simulink model "VCU_CS75_12_16_Test"  (R2014a)
settings: Solver=FixedStepDiscrete  StartTime=0.0  StopTime=25  FixedStep=0.0005  RelTol=1e-3
undefined symbols (not defined in the file): ecucoder_acal, I_SW01_L, LaterlAngleCommand, LDW, RemoteAcclPosition
libraries: simulink x913, ec5744lib x39
(part 30 of 30)

== system VCU_CS75_12_16_Test/长安CS75底盘程序，20ms一次/Input/CAN1_Rx/ESP_277/ReceiveMessages/Subsystem/ESP_1/ESP_AWBavailable_Sub ==
  In1 : Inport
  Out1 : Outport
  wires:
  In1/1 -> Out1/1

== system VCU_CS75_12_16_Test/长安CS75底盘程序，20ms一次/Input/CAN1_Rx/ESP_277/ReceiveMessages/Subsystem/ESP_1/ESP_BrakeForce_Sub ==
  In1 : Inport
  Out1 : Outport
  wires:
  In1/1 -> Out1/1

== system VCU_CS75_12_16_Test/长安CS75底盘程序，20ms一次/Input/CAN1_Rx/ESP_277/ReceiveMessages/Subsystem/ESP_1/ESP_BrakeOverHeat_Sub ==
  In1 : Inport
  Out1 : Outport
  wires:
  In1/1 -> Out1/1

== system VCU_CS75_12_16_Test/长安CS75底盘程序，20ms一次/Input/CAN1_Rx/ESP_277/ReceiveMessages/Subsystem/ESP_1/ESP_CDD_Active_APA_Sub ==
  In1 : Inport
  Out1 : Outport
  wires:
  In1/1 -> Out1/1

== system VCU_CS75_12_16_Test/长安CS75底盘程序，20ms一次/Input/CAN1_Rx/ESP_277/ReceiveMessages/Subsystem/ESP_1/ESP_CDD_Active_Sub ==
  In1 : Inport
  Out1 : Outport
  wires:
  In1/1 -> Out1/1

== system VCU_CS75_12_16_Test/长安CS75底盘程序，20ms一次/Input/CAN1_Rx/ESP_277/ReceiveMessages/Subsystem/ESP_1/ESP_CDD_Available_APA_Sub ==
  In1 : Inport
  Out1 : Outport
  wires:
  In1/1 -> Out1/1

== system VCU_CS75_12_16_Test/长安CS75底盘程序，20ms一次/Input/CAN1_Rx/ESP_277/ReceiveMessages/Subsystem/ESP_1/ESP_CDD_Available_Sub ==
  In1 : Inport
  Out1 : Outport
  wires:
  In1/1 -> Out1/1

== system VCU_CS75_12_16_Test/长安CS75底盘程序，20ms一次/Input/CAN1_Rx/ESP_277/ReceiveMessages/Subsystem/ESP_1/ESP_CheckSum_277_Sub ==
  In1 : Inport
  Out1 : Outport
  wires:
  In1/1 -> Out1/1

== system VCU_CS75_12_16_Test/长安CS75底盘程序，20ms一次/Input/CAN1_Rx/ESP_277/ReceiveMessages/Subsystem/ESP_1/ESP_PrefillActive_Sub ==
  In1 : Inport
  Out1 : Outport
  wires:
  In1/1 -> Out1/1

== system VCU_CS75_12_16_Test/长安CS75底盘程序，20ms一次/Input/CAN1_Rx/ESP_277/ReceiveMessages/Subsystem/ESP_1/ESP_PrefillAvailable_Sub ==
  In1 : Inport
  Out1 : Outport
  wires:
  In1/1 -> Out1/1

== system VCU_CS75_12_16_Test/长安CS75底盘程序，20ms一次/Input/CAN1_Rx/ESP_277/ReceiveMessages/Subsystem/ESP_1/ESP_RollingCounter_277_Sub ==
  In1 : Inport
  Out1 : Outport
  wires:
  In1/1 -> Out1/1

== system VCU_CS75_12_16_Test/长安CS75底盘程序，20ms一次/Input/CAN1_Rx/ESP_277/ReceiveMessages/Subsystem/ESP_1/ESP_TCSActive_Sub ==
  In1 : Inport
  Out1 : Outport
  wires:
  In1/1 -> Out1/1

== system VCU_CS75_12_16_Test/长安CS75底盘程序，20ms一次/Input/CAN1_Rx/ESP_277/ReceiveMessages/Subsystem/ESP_1/ESP_VDCActive_Sub ==
  In1 : Inport
  Out1 : Outport
  wires:
  In1/1 -> Out1/1

== system VCU_CS75_12_16_Test/长安CS75底盘程序，20ms一次/Input/CAN1_Rx/ESP_277/ReceiveMessages/Subsystem/ESP_1/ESP_VehicleStandstill_Sub ==
  In1 : Inport
  Out1 : Outport
  wires:
  In1/1 -> Out1/1

== system VCU_CS75_12_16_Test/长安CS75底盘程序，20ms一次/Input/CAN1_Rx/ESP_280/ReceiveMessages/Subsystem/ESP_1/Wheel_Speed_FL_Data_Sub ==
  In1 : Inport
  Out1 : Outport
  wires:
  In1/1 -> Out1/1

== system VCU_CS75_12_16_Test/长安CS75底盘程序，20ms一次/Input/CAN1_Rx/ESP_280/ReceiveMessages/Subsystem/ESP_1/Wheel_Speed_FL_Direction_Sub ==
  In1 : Inport
  Out1 : Outport
  wires:
  In1/1 -> Out1/1

== system VCU_CS75_12_16_Test/长安CS75底盘程序，20ms一次/Input/CAN1_Rx/ESP_280/ReceiveMessages/Subsystem/ESP_1/Wheel_Speed_FL_Valid_Data_Sub ==
  In1 : Inport
  Out1 : Outport
  wires:
  In1/1 -> Out1/1

== system VCU_CS75_12_16_Test/长安CS75底盘程序，20ms一次/Input/CAN1_Rx/ESP_280/ReceiveMessages/Subsystem/ESP_1/Wheel_Speed_FR_Data_Sub ==
  In1 : Inport
  Out1 : Outport
  wires:
  In1/1 -> Out1/1

== system VCU_CS75_12_16_Test/长安CS75底盘程序，20ms一次/Input/CAN1_Rx/ESP_280/ReceiveMessages/Subsystem/ESP_1/Wheel_Speed_FR_Direction_Sub ==
  In1 : Inport
  Out1 : Outport
  wires:
  In1/1 -> Out1/1

== system VCU_CS75_12_16_Test/长安CS75底盘程序，20ms一次/Input/CAN1_Rx/ESP_280/ReceiveMessages/Subsystem/ESP_1/Wheel_Speed_FR_Valid_Data_Sub ==
  In1 : Inport
  Out1 : Outport
  wires:
  In1/1 -> Out1/1

== system VCU_CS75_12_16_Test/长安CS75底盘程序，20ms一次/Input/CAN1_Rx/ESP_280/ReceiveMessages/Subsystem/ESP_1/Wheel_Speed_RL_Data_Sub ==
  In1 : Inport
  Out1 : Outport
  wires:
  In1/1 -> Out1/1

== system VCU_CS75_12_16_Test/长安CS75底盘程序，20ms一次/Input/CAN1_Rx/ESP_280/ReceiveMessages/Subsystem/ESP_1/Wheel_Speed_RL_Direction_Sub ==
  In1 : Inport
  Out1 : Outport
  wires:
  In1/1 -> Out1/1

== system VCU_CS75_12_16_Test/长安CS75底盘程序，20ms一次/Input/CAN1_Rx/ESP_280/ReceiveMessages/Subsystem/ESP_1/Wheel_Speed_RL_Valid_Data_Sub ==
  In1 : Inport
  Out1 : Outport
  wires:
  In1/1 -> Out1/1

== system VCU_CS75_12_16_Test/长安CS75底盘程序，20ms一次/Input/CAN1_Rx/ESP_280/ReceiveMessages/Subsystem/ESP_1/Wheel_Speed_RR_Data_Sub ==
  In1 : Inport
  Out1 : Outport
  wires:
  In1/1 -> Out1/1

== system VCU_CS75_12_16_Test/长安CS75底盘程序，20ms一次/Input/CAN1_Rx/ESP_280/ReceiveMessages/Subsystem/ESP_1/Wheel_Speed_RR_Direction_Sub ==
  In1 : Inport
  Out1 : Outport
  wires:
  In1/1 -> Out1/1

== system VCU_CS75_12_16_Test/长安CS75底盘程序，20ms一次/Input/CAN1_Rx/ESP_280/ReceiveMessages/Subsystem/ESP_1/Wheel_Speed_RR_Valid_Data_Sub ==
  In1 : Inport
  Out1 : Outport
  wires:
  In1/1 -> Out1/1

== system VCU_CS75_12_16_Test/长安CS75底盘程序，20ms一次/Input/CAN1_Rx/ESP_281/ReceiveMessages/Subsystem/ESP_2/ESP_ABSActiveStatus_Sub ==
  In1 : Inport
  Out1 : Outport
  wires:
  In1/1 -> Out1/1

== system VCU_CS75_12_16_Test/长安CS75底盘程序，20ms一次/Input/CAN1_Rx/ESP_281/ReceiveMessages/Subsystem/ESP_2/ESP_ABSFailStatus_Sub ==
  In1 : Inport
  Out1 : Outport
  wires:
  In1/1 -> Out1/1

== system VCU_CS75_12_16_Test/长安CS75底盘程序，20ms一次/Input/CAN1_Rx/ESP_281/ReceiveMessages/Subsystem/ESP_2/ESP_BrakePedalStatus_Sub ==
  In1 : Inport
  Out1 : Outport
  wires:
  In1/1 -> Out1/1

== system VCU_CS75_12_16_Test/长安CS75底盘程序，20ms一次/Input/CAN1_Rx/ESP_281/ReceiveMessages/Subsystem/ESP_2/ESP_Checksum_Sub ==
  In1 : Inport
  Out1 : Outport
  wires:
  In1/1 -> Out1/1

== system VCU_CS75_12_16_Test/长安CS75底盘程序，20ms一次/Input/CAN1_Rx/ESP_281/ReceiveMessages/Subsystem/ESP_2/ESP_EBDFailStatus_Sub ==
  In1 : Inport
  Out1 : Outport
  wires:
  In1/1 -> Out1/1

== system VCU_CS75_12_16_Test/长安CS75底盘程序，20ms一次/Input/CAN1_Rx/ESP_281/ReceiveMessages/Subsystem/ESP_2/ESP_ESPActiveStatus_Sub ==
  In1 : Inport
  Out1 : Outport
  wires:
  In1/1 -> Out1/1

== system VCU_CS75_12_16_Test/长安CS75底盘程序，20ms一次/Input/CAN1_Rx/ESP_281/ReceiveMessages/Subsystem/ESP_2/ESP_ESPFailStatus_Sub ==
  In1 : Inport
  Out1 : Outport
  wires:
  In1/1 -> Out1/1

== system VCU_CS75_12_16_Test/长安CS75底盘程序，20ms一次/Input/CAN1_Rx/ESP_281/ReceiveMessages/Subsystem/ESP_2/ESP_ESPSwitchStatus_Sub ==
  In1 : Inport
  Out1 : Outport
  wires:
  In1/1 -> Out1/1

== system VCU_CS75_12_16_Test/长安CS75底盘程序，20ms一次/Input/CAN1_Rx/ESP_281/ReceiveMessages/Subsystem/ESP_2/ESP_RollingCounter_Sub ==
  In1 : Inport
  Out1 : Outport
  wires:
  In1/1 -> Out1/1

== system VCU_CS75_12_16_Test/长安CS75底盘程序，20ms一次/Input/CAN1_Rx/ESP_281/ReceiveMessages/Subsystem/ESP_2/ESP_VehicleSpeed_Status_Sub ==
  In1 : Inport
  Out1 : Outport
  wires:
  In1/1 -> Out1/1

== system VCU_CS75_12_16_Test/长安CS75底盘程序，20ms一次/Input/CAN1_Rx/ESP_281/ReceiveMessages/Subsystem/ESP_2/ESP_VehicleSpeed_Sub ==
  In1 : Inport
  Out1 : Outport
  wires:
  In1/1 -> Out1/1

== system VCU_CS75_12_16_Test/长安CS75底盘程序，20ms一次/Input/CAN1_Rx/ESP_287/ReceiveMessages/Subsystem/ESP_2/ESP_CheckSum_Sub ==
  In1 : Inport
  Out1 : Outport
  wires:
  In1/1 -> Out1/1

== system VCU_CS75_12_16_Test/长安CS75底盘程序，20ms一次/Input/CAN1_Rx/ESP_287/ReceiveMessages/Subsystem/ESP_2/ESP_HBBActiveStatus_Sub ==
  In1 : Inport
  Out1 : Outport
  wires:
  In1/1 -> Out1/1

== system VCU_CS75_12_16_Test/长安CS75底盘程序，20ms一次/Input/CAN1_Rx/ESP_287/ReceiveMessages/Subsystem/ESP_2/ESP_HBB_Status_Sub ==
  In1 : Inport
  Out1 : Outport
  wires:
  In1/1 -> Out1/1

== system VCU_CS75_12_16_Test/长安CS75底盘程序，20ms一次/Input/CAN1_Rx/ESP_287/ReceiveMessages/Subsystem/ESP_2/ESP_HDC_Status_Sub ==
  In1 : Inport
  Out1 : Outport
  wires:
  In1/1 -> Out1/1

== system VCU_CS75_12_16_Test/长安CS75底盘程序，20ms一次/Input/CAN1_Rx/ESP_287/ReceiveMessages/Subsystem/ESP_2/ESP_HHC_Available_Sub ==
  In1 : Inport
  Out1 : Outport
  wires:
  In1/1 -> Out1/1

== system VCU_CS75_12_16_Test/长安CS75底盘程序，20ms一次/Input/CAN1_Rx/ESP_287/ReceiveMessages/Subsystem/ESP_2/ESP_LatAcceleration_Sub ==
  In1 : Inport
  Out1 : Outport
  wires:
  In1/1 -> Out1/1

== system VCU_CS75_12_16_Test/长安CS75底盘程序，20ms一次/Input/CAN1_Rx/ESP_287/ReceiveMessages/Subsystem/ESP_2/ESP_LongAccelValid_Sub ==
  In1 : Inport
  Out1 : Outport
  wires:
  In1/1 -> Out1/1

== system VCU_CS75_12_16_Test/长安CS75底盘程序，20ms一次/Input/CAN1_Rx/ESP_287/ReceiveMessages/Subsystem/ESP_2/ESP_LongAcceleration_Sub ==
  In1 : Inport
  Out1 : Outport
  wires:
  In1/1 -> Out1/1

== system VCU_CS75_12_16_Test/长安CS75底盘程序，20ms一次/Input/CAN1_Rx/ESP_287/ReceiveMessages/Subsystem/ESP_2/ESP_RollingCounter_Sub ==
  In1 : Inport
  Out1 : Outport
  wires:
  In1/1 -> Out1/1

== system VCU_CS75_12_16_Test/长安CS75底盘程序，20ms一次/Input/CAN1_Rx/ESP_287/ReceiveMessages/Subsystem/ESP_2/ESP_TODFastOpenRequest_Sub ==
  In1 : Inport
  Out1 : Outport
  wires:
  In1/1 -> Out1/1

== system VCU_CS75_12_16_Test/长安CS75底盘程序，20ms一次/Input/CAN1_Rx/ESP_287/ReceiveMessages/Subsystem/ESP_2/ESP_TODTorqueMaxLimit_Sub ==
  In1 : Inport
  Out1 : Outport
  wires:
  In1/1 -> Out1/1

== system VCU_CS75_12_16_Test/长安CS75底盘程序，20ms一次/Input/CAN1_Rx/ESP_287/ReceiveMessages/Subsystem/ESP_2/ESP_YawRate_Status_Sub ==
  In1 : Inport
  Out1 : Outport
  wires:
  In1/1 -> Out1/1

== system VCU_CS75_12_16_Test/长安CS75底盘程序，20ms一次/Input/CAN1_Rx/ESP_287/ReceiveMessages/Subsystem/ESP_2/ESP_YawRate_Sub ==
  In1 : Inport
  Out1 : Outport
  wires:
  In1/1 -> Out1/1

== system VCU_CS75_12_16_Test/长安CS75底盘程序，20ms一次/Input/CAN1_Rx/GW_20B/ReceiveMessages/Subsystem/GW_20B2/EMS_BrakePedalStatus_Sub ==
  In1 : Inport
  Out1 : Outport
  wires:
  In1/1 -> Out1/1

== system VCU_CS75_12_16_Test/长安CS75底盘程序，20ms一次/Input/CAN1_Rx/GW_20B/ReceiveMessages/Subsystem/GW_20B2/EMS_EngineStartupEnd_Sub ==
  In1 : Inport
  Out1 : Outport
  wires:
  In1/1 -> Out1/1

== system VCU_CS75_12_16_Test/长安CS75底盘程序，20ms一次/Input/CAN1_Rx/GW_20B/ReceiveMessages/Subsystem/GW_20B2/EMS_EngineStatus_Sub ==
  In1 : Inport
  Out1 : Outport
  wires:
  In1/1 -> Out1/1

== system VCU_CS75_12_16_Test/长安CS75底盘程序，20ms一次/Input/CAN1_Rx/GW_20B/ReceiveMessages/Subsystem/GW_20B2/EPB_BrakeLightOnRequest_Sub ==
  In1 : Inport
  Out1 : Outport
  wires:
  In1/1 -> Out1/1

== system VCU_CS75_12_16_Test/长安CS75底盘程序，20ms一次/Input/CAN1_Rx/GW_20B/ReceiveMessages/Subsystem/GW_20B2/EPB_Status_Sub ==
  In1 : Inport
  Out1 : Outport
  wires:
  In1/1 -> Out1/1

== system VCU_CS75_12_16_Test/长安CS75底盘程序，20ms一次/Input/CAN1_Rx/GW_20B/ReceiveMessages/Subsystem/GW_20B2/SAS_SteeringAngleValid_Sub ==
  In1 : Inport
  Out1 : Outport
  wires:
  In1/1 -> Out1/1

== system VCU_CS75_12_16_Test/长安CS75底盘程序，20ms一次/Input/CAN1_Rx/GW_20B/ReceiveMessages/Subsystem/GW_20B2/SAS_SteeringAngle_Sub ==
  In1 : Inport
  Out1 : Outport
  wires:
  In1/1 -> Out1/1

== system VCU_CS75_12_16_Test/长安CS75底盘程序，20ms一次/Input/CAN1_Rx/GW_20B/ReceiveMessages/Subsystem/GW_20B2/TCU_GearShiftPositon_Sub ==
  In1 : Inport
  Out1 : Outport
  wires:
  In1/1 -> Out1/1

== system VCU_CS75_12_16_Test/长安CS75底盘程序，20ms一次/Input/CAN1_Rx/GW_20B/ReceiveMessages/Subsystem/GW_20B2/TCU_ShiftPostionValid_Sub ==
  In1 : Inport
  Out1 : Outport
  wires:
  In1/1 -> Out1/1

== system VCU_CS75_12_16_Test/长安CS75底盘程序，20ms一次/Input/CAN1_Rx/GW_308/ReceiveMessages/Subsystem/GW_1/IP_TotalOdometer_Sub ==
  In1 : Inport
  Out1 : Outport
  wires:
  In1/1 -> Out1/1

== system VCU_CS75_12_16_Test/长安CS75底盘程序，20ms一次/Input/CAN1_Rx/GW_332/ReceiveMessages/Subsystem/GW_1/EMS_EngineSpeed_Sub ==
  In1 : Inport
  Out1 : Outport
  wires:
  In1/1 -> Out1/1

== system VCU_CS75_12_16_Test/长安CS75底盘程序，20ms一次/Input/CAN1_Rx/GW_332/ReceiveMessages/Subsystem/GW_1/SAS_SASFailure_Sub ==
  In1 : Inport
  Out1 : Outport
  wires:
  In1/1 -> Out1/1

== system VCU_CS75_12_16_Test/长安CS75底盘程序，20ms一次/Input/CAN1_Rx/GW_332/ReceiveMessages/Subsystem/GW_1/SRS_DriverBuckleSwitchStatus_Sub ==
  In1 : Inport
  Out1 : Outport
  wires:
  In1/1 -> Out1/1

== system VCU_CS75_12_16_Test/长安CS75底盘程序，20ms一次/Input/CAN1_Rx/GW_332/ReceiveMessages/Subsystem/GW_1/SRS_PassengerBuckleSwitchStatus_Sub ==
  In1 : Inport
  Out1 : Outport
  wires:
  In1/1 -> Out1/1

== system VCU_CS75_12_16_Test/长安CS75底盘程序，20ms一次/Input/CAN1_Rx/GW_376/ReceiveMessages/Subsystem/GW_2/EMS_ConditionIdle_Sub ==
  In1 : Inport
  Out1 : Outport
  wires:
  In1/1 -> Out1/1

== system VCU_CS75_12_16_Test/长安CS75底盘程序，20ms一次/Input/CAN1_Rx/GW_376/ReceiveMessages/Subsystem/GW_2/EMS_EngineFuelCutOff_Sub ==
  In1 : Inport
  Out1 : Outport
  wires:
  In1/1 -> Out1/1

== system VCU_CS75_12_16_Test/长安CS75底盘程序，20ms一次/Input/CAN1_Rx/GW_376/ReceiveMessages/Subsystem/GW_2/EMS_FrictionalTorq_Sub ==
  In1 : Inport
  Out1 : Outport
  wires:
  In1/1 -> Out1/1

== system VCU_CS75_12_16_Test/长安CS75底盘程序，20ms一次/Input/CAN1_Rx/GW_376/ReceiveMessages/Subsystem/GW_2/EMS_TorqueConstant_Sub ==
  In1 : Inport
  Out1 : Outport
  wires:
  In1/1 -> Out1/1

== system VCU_CS75_12_16_Test/长安CS75底盘程序，20ms一次/Input/CAN1_Rx/GW_3A2/ReceiveMessages/Subsystem/GW_3A1/ACC_ACCMode_Sub ==
  In1 : Inport
  Out1 : Outport
  wires:
  In1/1 -> Out1/1

== system VCU_CS75_12_16_Test/长安CS75底盘程序，20ms一次/Input/CAN1_Rx/GW_3A2/ReceiveMessages/Subsystem/GW_3A1/EMS_RemindGear_Sub ==
  In1 : Inport
  Out1 : Outport
  wires:
  In1/1 -> Out1/1

== system VCU_CS75_12_16_Test/长安CS75底盘程序，20ms一次/Input/CAN1_Rx/GW_3A2/ReceiveMessages/Subsystem/GW_3A1/EMS_RemindShiftGear_Sub ==
  In1 : Inport
  Out1 : Outport
  wires:
  In1/1 -> Out1/1

== system VCU_CS75_12_16_Test/长安CS75底盘程序，20ms一次/Input/CAN1_Rx/GW_3A2/ReceiveMessages/Subsystem/GW_3A1/EPB_FunctionLamp_Sub ==
  In1 : Inport
  Out1 : Outport
  wires:
  In1/1 -> Out1/1

== system VCU_CS75_12_16_Test/长安CS75底盘程序，20ms一次/Input/CAN1_Rx/GW_3A2/ReceiveMessages/Subsystem/GW_3A1/EPB_SwitchPositionValid_Sub ==
  In1 : Inport
  Out1 : Outport
  wires:
  In1/1 -> Out1/1

== system VCU_CS75_12_16_Test/长安CS75底盘程序，20ms一次/Input/CAN1_Rx/GW_3A2/ReceiveMessages/Subsystem/GW_3A1/EPB_SwitchPosition_Sub ==
  In1 : Inport
  Out1 : Outport
  wires:
  In1/1 -> Out1/1

== system VCU_CS75_12_16_Test/长安CS75底盘程序，20ms一次/Input/CAN1_Rx/GW_3A2/ReceiveMessages/Subsystem/GW_3A1/EPB_TextDisplay_Sub ==
  In1 : Inport
  Out1 : Outport
  wires:
  In1/1 -> Out1/1

== system VCU_CS75_12_16_Test/长安CS75底盘程序，20ms一次/Input/CAN1_Rx/GW_3A2/ReceiveMessages/Subsystem/GW_3A1/EPS_EPSFailed_Sub ==
  In1 : Inport
  Out1 : Outport
  wires:
  In1/1 -> Out1/1

== system VCU_CS75_12_16_Test/长安CS75底盘程序，20ms一次/Input/CAN1_Rx/GW_3A2/ReceiveMessages/Subsystem/GW_3A1/EPS_TorqueAssistMode_Sub ==
  In1 : Inport
  Out1 : Outport
  wires:
  In1/1 -> Out1/1

== system VCU_CS75_12_16_Test/长安CS75底盘程序，20ms一次/Input/CAN1_Rx/GW_3A2/ReceiveMessages/Subsystem/GW_3A1/ESP_AutoHoldActive_Sub ==
  In1 : Inport
  Out1 : Outport
  wires:
  In1/1 -> Out1/1

== system VCU_CS75_12_16_Test/长安CS75底盘程序，20ms一次/Input/CAN1_Rx/GW_3A2/ReceiveMessages/Subsystem/GW_3A1/ESP_AutoHoldAvailable_Sub ==
  In1 : Inport
  Out1 : Outport
  wires:
  In1/1 -> Out1/1

== system VCU_CS75_12_16_Test/长安CS75底盘程序，20ms一次/Input/CAN1_Rx/GW_3A2/ReceiveMessages/Subsystem/GW_3A1/ESP_EBDFailStatus_Sub ==
  In1 : Inport
  Out1 : Outport
  wires:
  In1/1 -> Out1/1

== system VCU_CS75_12_16_Test/长安CS75底盘程序，20ms一次/Input/CAN1_Rx/GW_3A2/ReceiveMessages/Subsystem/GW_3A1/ESP_ESPActiveStatus_Sub ==
  In1 : Inport
  Out1 : Outport
  wires:
  In1/1 -> Out1/1

== system VCU_CS75_12_16_Test/长安CS75底盘程序，20ms一次/Input/CAN1_Rx/GW_3A2/ReceiveMessages/Subsystem/GW_3A1/ESP_ESPFunctionStatus_Sub ==
  In1 : Inport
  Out1 : Outport
  wires:
  In1/1 -> Out1/1

== system VCU_CS75_12_16_Test/长安CS75底盘程序，20ms一次/Input/CAN1_Rx/GW_3A2/ReceiveMessages/Subsystem/GW_3A1/ESP_HBBFunctionStatus_Sub ==
  In1 : Inport
  Out1 : Outport
  wires:
  In1/1 -> Out1/1

== system VCU_CS75_12_16_Test/长安CS75底盘程序，20ms一次/Input/CAN1_Rx/GW_3A2/ReceiveMessages/Subsystem/GW_3A1/ESP_HDC_STATUS_Sub ==
  In1 : Inport
  Out1 : Outport
  wires:
  In1/1 -> Out1/1

== system VCU_CS75_12_16_Test/长安CS75底盘程序，20ms一次/Input/CAN1_Rx/GW_3A2/ReceiveMessages/Subsystem/GW_3A1/ESP_HHC_Active_Sub ==
  In1 : Inport
  Out1 : Outport
  wires:
  In1/1 -> Out1/1

== system VCU_CS75_12_16_Test/长安CS75底盘程序，20ms一次/Input/CAN1_Rx/GW_3A2/ReceiveMessages/Subsystem/GW_3A1/ESP_HHC_Available_Sub ==
  In1 : Inport
  Out1 : Outport
  wires:
  In1/1 -> Out1/1

== system VCU_CS75_12_16_Test/长安CS75底盘程序，20ms一次/Input/CAN1_Rx/GW_3A2/ReceiveMessages/Subsystem/GW_3A1/SRS_LeftRearBuckleSwitchSts_Sub ==
  In1 : Inport
  Out1 : Outport
  wires:
  In1/1 -> Out1/1

== system VCU_CS75_12_16_Test/长安CS75底盘程序，20ms一次/Input/CAN1_Rx/GW_3A2/ReceiveMessages/Subsystem/GW_3A1/SRS_MiddleRearBuckleSwitchSts_Sub ==
  In1 : Inport
  Out1 : Outport
  wires:
  In1/1 -> Out1/1

== system VCU_CS75_12_16_Test/长安CS75底盘程序，20ms一次/Input/CAN1_Rx/GW_3A2/ReceiveMessages/Subsystem/GW_3A1/SRS_RightRearBuckleSwitchSts_Sub ==
  In1 : Inport
  Out1 : Outport
  wires:
  In1/1 -> Out1/1

== system VCU_CS75_12_16_Test/长安CS75底盘程序，20ms一次/Input/CAN1_Rx/GW_3A2/ReceiveMessages/Subsystem/GW_3A1/TCU_FailureLamp_Sub ==
  In1 : Inport
  Out1 : Outport
  wires:
  In1/1 -> Out1/1

== system VCU_CS75_12_16_Test/长安CS75底盘程序，20ms一次/Input/CAN1_Rx/GW_3A2/ReceiveMessages/Subsystem/GW_3A1/TCU_GearForDisplay_Sub ==
  In1 : Inport
  Out1 : Outport
  wires:
  In1/1 -> Out1/1

== system VCU_CS75_12_16_Test/长安CS75底盘程序，20ms一次/Input/CAN1_Rx/GW_3A2/ReceiveMessages/Subsystem/GW_3A1/TCU_GearIndication_Sub ==
  In1 : Inport
  Out1 : Outport
  wires:
  In1/1 -> Out1/1

== system VCU_CS75_12_16_Test/长安CS75底盘程序，20ms一次/Input/CAN1_Rx/GW_3A2/ReceiveMessages/Subsystem/GW_3A1/TCU_PWRLamp_Sub ==
  In1 : Inport
  Out1 : Outport
  wires:
  In1/1 -> Out1/1

== system VCU_CS75_12_16_Test/长安CS75底盘程序，20ms一次/Input/CAN1_Rx/GW_3A2/ReceiveMessages/Subsystem/GW_3A1/TCU_ReqTranTempWarning_Sub ==
  In1 : Inport
  Out1 : Outport
  wires:
  In1/1 -> Out1/1

== system VCU_CS75_12_16_Test/长安CS75底盘程序，20ms一次/Input/CAN1_Rx/GW_3A2/ReceiveMessages/Subsystem/GW_3A1/TCU_WNTLamp_Sub ==
  In1 : Inport
  Out1 : Outport
  wires:
  In1/1 -> Out1/1

== system VCU_CS75_12_16_Test/长安CS75底盘程序，20ms一次/Input/CAN1_Rx/GW_567/ReceiveMessages/Subsystem/GW_2/HU_Byroad_Sub ==
  In1 : Inport
  Out1 : Outport
  wires:
  In1/1 -> Out1/1

== system VCU_CS75_12_16_Test/长安CS75底盘程序，20ms一次/Input/CAN1_Rx/GW_567/ReceiveMessages/Subsystem/GW_2/HU_EnterTunnelInfo_Sub ==
  In1 : Inport
  Out1 : Outport
  wires:
  In1/1 -> Out1/1

== system VCU_CS75_12_16_Test/长安CS75底盘程序，20ms一次/Input/CAN1_Rx/GW_567/ReceiveMessages/Subsystem/GW_2/HU_NavGuiganceStatus_Sub ==
  In1 : Inport
  Out1 : Outport
  wires:
  In1/1 -> Out1/1

== system VCU_CS75_12_16_Test/长安CS75底盘程序，20ms一次/Input/CAN1_Rx/GW_567/ReceiveMessages/Subsystem/GW_2/HU_TunnelDistance_Sub ==
  In1 : Inport
  Out1 : Outport
  wires:
  In1/1 -> Out1/1

== system VCU_CS75_12_16_Test/长安CS75底盘程序，20ms一次/Input/CAN1_Rx/GW_567/ReceiveMessages/Subsystem/GW_2/HU_TunnelLength_Sub ==
  In1 : Inport
  Out1 : Outport
  wires:
  In1/1 -> Out1/1

== system VCU_CS75_12_16_Test/长安CS75底盘程序，20ms一次/Input/CAN1_Rx/HU_GPS_500/ReceiveMessages/Subsystem/HU_GPS_1/GPSCurrentLocationValid_Sub ==
  In1 : Inport
  Out1 : Outport
  wires:
  In1/1 -> Out1/1

== system VCU_CS75_12_16_Test/长安CS75底盘程序，20ms一次/Input/CAN1_Rx/LAS_36E/ReceiveMessages/Subsystem/LAS_36E2/LAS_CheckSum_id36E_Sub ==
  In1 : Inport
  Out1 : Outport
  wires:
  In1/1 -> Out1/1

== system VCU_CS75_12_16_Test/长安CS75底盘程序，20ms一次/Input/CAN1_Rx/LAS_36E/ReceiveMessages/Subsystem/LAS_36E2/LAS_LaneEquationC1_Sub ==
  In1 : Inport
  Out1 : Outport
  wires:
  In1/1 -> Out1/1

== system VCU_CS75_12_16_Test/长安CS75底盘程序，20ms一次/Input/CAN1_Rx/LAS_36E/ReceiveMessages/Subsystem/LAS_36E2/LAS_LaneEquationC3_Sub ==
  In1 : Inport
  Out1 : Outport
  wires:
  In1/1 -> Out1/1

== system VCU_CS75_12_16_Test/长安CS75底盘程序，20ms一次/Input/CAN1_Rx/LAS_36E/ReceiveMessages/Subsystem/LAS_36E2/LAS_LaneEquationStatus_Sub ==
  In1 : Inport
  Out1 : Outport
  wires:
  In1/1 -> Out1/1

== system VCU_CS75_12_16_Test/长安CS75底盘程序，20ms一次/Input/CAN1_Rx/LAS_36E/ReceiveMessages/Subsystem/LAS_36E2/LAS_RoadCurvatureFar_Sub ==
  In1 : Inport
  Out1 : Outport
  wires:
  In1/1 -> Out1/1

== system VCU_CS75_12_16_Test/长安CS75底盘程序，20ms一次/Input/CAN1_Rx/LAS_36E/ReceiveMessages/Subsystem/LAS_36E2/LAS_RoadCurvatureNear_Sub ==
  In1 : Inport
  Out1 : Outport
  wires:
  In1/1 -> Out1/1

== system VCU_CS75_12_16_Test/长安CS75底盘程序，20ms一次/Input/CAN1_Rx/LAS_36E/ReceiveMessages/Subsystem/LAS_36E2/LAS_RollingCounter_id36E_Sub ==
  In1 : Inport
  Out1 : Outport
  wires:
  In1/1 -> Out1/1

== system VCU_CS75_12_16_Test/长安CS75底盘程序，20ms一次/Input/CAN1_Rx/SAS_108/ReceiveMessages/Subsystem/SAS_2/SAS_CRCCheck_Sub ==
  In1 : Inport
  Out1 : Outport
  wires:
  In1/1 -> Out1/1

== system VCU_CS75_12_16_Test/长安CS75底盘程序，20ms一次/Input/CAN1_Rx/SAS_108/ReceiveMessages/Subsystem/SAS_2/SAS_Calibrated_Sub ==
  In1 : Inport
  Out1 : Outport
  wires:
  In1/1 -> Out1/1

== system VCU_CS75_12_16_Test/长安CS75底盘程序，20ms一次/Input/CAN1_Rx/SAS_108/ReceiveMessages/Subsystem/SAS_2/SAS_RollingCounter_Sub ==
  In1 : Inport
  Out1 : Outport
  wires:
  In1/1 -> Out1/1

== system VCU_CS75_12_16_Test/长安CS75底盘程序，20ms一次/Input/CAN1_Rx/SAS_108/ReceiveMessages/Subsystem/SAS_2/SAS_SASFailure_Sub ==
  In1 : Inport
  Out1 : Outport
  wires:
  In1/1 -> Out1/1

== system VCU_CS75_12_16_Test/长安CS75底盘程序，20ms一次/Input/CAN1_Rx/SAS_108/ReceiveMessages/Subsystem/SAS_2/SAS_SteeringAngleSpeed_Sub ==
  In1 : Inport
  Out1 : Outport
  wires:
  In1/1 -> Out1/1

== system VCU_CS75_12_16_Test/长安CS75底盘程序，20ms一次/Input/CAN1_Rx/SAS_108/ReceiveMessages/Subsystem/SAS_2/SAS_SteeringAngleValid_Sub ==
  In1 : Inport
  Out1 : Outport
  wires:
  In1/1 -> Out1/1

== system VCU_CS75_12_16_Test/长安CS75底盘程序，20ms一次/Input/CAN1_Rx/SAS_108/ReceiveMessages/Subsystem/SAS_2/SAS_SteeringAngle_Sub ==
  In1 : Inport
  Out1 : Outport
  wires:
  In1/1 -> Out1/1

== system VCU_CS75_12_16_Test/长安CS75底盘程序，20ms一次/Input/CAN1_Rx/SCM_3B8/ReceiveMessages/Subsystem/SCM_3B2/SCM_ACCCancel_Sub ==
  In1 : Inport
  Out1 : Outport
  wires:
  In1/1 -> Out1/1

== system VCU_CS75_12_16_Test/长安CS75底盘程序，20ms一次/Input/CAN1_Rx/SCM_3B8/ReceiveMessages/Subsystem/SCM_3B2/SCM_ACCOn_Sub ==
  In1 : Inport
  Out1 : Outport
  wires:
  In1/1 -> Out1/1

== system VCU_CS75_12_16_Test/长安CS75底盘程序，20ms一次/Input/CAN1_Rx/SCM_3B8/ReceiveMessages/Subsystem/SCM_3B2/SCM_IACCOn_Sub ==
  In1 : Inport
  Out1 : Outport
  wires:
  In1/1 -> Out1/1

== system VCU_CS75_12_16_Test/长安CS75底盘程序，20ms一次/Input/CAN1_Rx/SCM_3B8/ReceiveMessages/Subsystem/SCM_3B2/SCM_Resume_Sub ==
  In1 : Inport
  Out1 : Outport
  wires:
  In1/1 -> Out1/1

== system VCU_CS75_12_16_Test/长安CS75底盘程序，20ms一次/Input/CAN1_Rx/SCM_3B8/ReceiveMessages/Subsystem/SCM_3B2/SCM_Speeddecrease_Sub ==
  In1 : Inport
  Out1 : Outport
  wires:
  In1/1 -> Out1/1

== system VCU_CS75_12_16_Test/长安CS75底盘程序，20ms一次/Input/CAN1_Rx/SCM_3B8/ReceiveMessages/Subsystem/SCM_3B2/SCM_TimeGap_Sub ==
  In1 : Inport
  Out1 : Outport
  wires:
  In1/1 -> Out1/1

== system VCU_CS75_12_16_Test/长安CS75底盘程序，20ms一次/Input/CAN1_Rx/SRS_005/ReceiveMessages/Subsystem/SRS_1/SRS_DriverBuckleSwitchStatus_Sub ==
  In1 : Inport
  Out1 : Outport
  wires:
  In1/1 -> Out1/1

== system VCU_CS75_12_16_Test/长安CS75底盘程序，20ms一次/Input/CAN1_Rx/SRS_005/ReceiveMessages/Subsystem/SRS_1/SRS_RollingCounter_Sub ==
  In1 : Inport
  Out1 : Outport
  wires:
  In1/1 -> Out1/1

== system VCU_CS75_12_16_Test/长安CS75底盘程序，20ms一次/Input/CAN1_Rx/TCU_286/ReceiveMessages/Subsystem/TCU_1/TCU_ActualGearValid_Sub ==
  In1 : Inport
  Out1 : Outport
  wires:
  In1/1 -> Out1/1

== system VCU_CS75_12_16_Test/长安CS75底盘程序，20ms一次/Input/CAN1_Rx/TCU_286/ReceiveMessages/Subsystem/TCU_1/TCU_ActualGear_Sub ==
  In1 : Inport
  Out1 : Outport
  wires:
  In1/1 -> Out1/1

== system VCU_CS75_12_16_Test/长安CS75底盘程序，20ms一次/Input/CAN1_Rx/TCU_286/ReceiveMessages/Subsystem/TCU_1/TCU_GearShiftPosition_Sub ==
  In1 : Inport
  Out1 : Outport
  wires:
  In1/1 -> Out1/1

== system VCU_CS75_12_16_Test/长安CS75底盘程序，20ms一次/Input/CAN1_Rx/TCU_286/ReceiveMessages/Subsystem/TCU_1/TCU_ShiftPositionValid_Sub ==
  In1 : Inport
  Out1 : Outport
  wires:
  In1/1 -> Out1/1

== matlab function VCU_CS75_12_16_Test/长安CS75底盘程序，20ms一次/APP/Controller/Lateral/MATLAB Function3 ==
  data: LAS_Status output; P6 input; LateralTakeover output; System_State input
function [LAS_Status,LateralTakeover]   = fcn(P6,System_State)
if P6 == 1 && (System_State == 0 || System_State == 1)
     LateralTakeover = 1;
     LAS_Status = 2;
else
     LateralTakeover = 0;
     LAS_Status = 1;
end  
end

== matlab function VCU_CS75_12_16_Test/长安CS75底盘程序，20ms一次/APP/Monitor/Vehicle_Status/MATLAB Function4 ==
  data: TimeThreshold input; EPS_CommunicationStatus output; RollingCounter input; LastRollingCounter input; LastCounter input; Counter output
function [EPS_CommunicationStatus,Counter]  = fcn(TimeThreshold,RollingCounter,LastRollingCounter,LastCounter)
if RollingCounter == LastRollingCounter
    Counter = LastCounter + 1;
else
    Counter = 0;
end
if (Counter * 20) > TimeThreshold
    EPS_CommunicationStatus = 0;
else
    EPS_CommunicationStatus = 1;
end
end

== matlab function VCU_CS75_12_16_Test/长安CS75底盘程序，20ms一次/APP/Monitor/Server_Status/MATLAB Function1 ==
  data: TimeThreshold input; EPS_CommunicationStatus output; RollingCounter input; LastRollingCounter input; LastCounter input; Counter output
function [EPS_CommunicationStatus,Counter]  = fcn(TimeThreshold,RollingCounter,LastRollingCounter,LastCounter)
if RollingCounter == LastRollingCounter
    Counter = LastCounter + 1;
else
    Counter = 0;
end
if (Counter * 20) > TimeThreshold
    EPS_CommunicationStatus = 0;
else
    EPS_CommunicationStatus = 1;
end
end

== stateflow chart VCU_CS75_12_16_Test/长安CS75底盘程序，20ms一次/APP/System_State_Manager/Chart ==
  state System_State
    state INIT_ManualDriving
      %驾驶员正常驾驶
      en,du:
      System_State = 0;
    state TakeOver
      %人工接管模式
      en,du:
      System_State = 2;
    state AutoDriving
      %自动驾驶
      en,du:
      System_State = 1;
    state Error
      %故障，需人工接管
      en,du:
      System_State = 3;
    (default) -> INIT_ManualDriving
    INIT_ManualDriving -> AutoDriving : [AutoDrivingReady == 1&& Server_CommunicationStatus == 1 && TakeoverStatus == 0 && VehicleComminicationStatus == 1 && VehicleFaultStatus == 0 ]%% &&Switch_P6 == 1&&EPS_AvailabilityStatus == 2
    Error -> INIT_ManualDriving : [AutoDrivingReady == 0 &&Switch_P6 == 0 && VehicleComminicationStatus == 1&& VehicleFaultStatus == 0]%%&& Server_CommunicationStatus == 1
    AutoDriving -> INIT_ManualDriving [order 3] : [AutoDrivingReady == 0 ]%%&&Switch_P6 == 0
    TakeOver -> INIT_ManualDriving [order 1] : [AutoDrivingReady == 0 && Switch_P6 == 0]
    AutoDriving -> TakeOver [order 2] : [TakeoverStatus == 1]
    AutoDriving -> Error [order 1] : [VehicleFaultStatus == 1 || VehicleComminicationStatus == 0 || Server_CommunicationStatus ==0]
    TakeOver -> Error [order 2] : [VehicleFaultStatus == 1 || VehicleComminicationStatus == 0 || Server_CommunicationStatus ==0]
  data: VehicleFaultStatus input; VehicleComminicationStatus input; EPS_AvailabilityStatus input; TakeoverStatus input; Server_CommunicationStatus input; AutoDrivingReady input; System_State output; Switch_P6 input

== matlab function VCU_CS75_12_16_Test/长安CS75底盘程序，20ms一次/APP/Controller/General/MATLAB Function ==
  data: u input; y output
function y = fcn(u)
if u == 1
    y = 1;
else
    y = 0;
end
end

== matlab function VCU_CS75_12_16_Test/长安CS75底盘程序，20ms一次/APP/Controller/Longitudinal/MATLAB Function ==
  data: u input; y output
function y = fcn(u)
if u < 0
    y = 1;
else
    y = 0;
end
end

== matlab function VCU_CS75_12_16_Test/长安CS75底盘程序，20ms一次/APP/Controller/Longitudinal/MATLAB Function1 ==
  data: u input; y output
function y = fcn(u)
if u >= 0
    y = 1;
else
    y = 0;
end
end

== matlab function VCU_CS75_12_16_Test/长安CS75底盘程序，20ms一次/APP/Controller/Longitudinal/MATLAB Function2 ==
  data: u1 input; y output; u2 input
function y = fcn(u1,u2)
if u1 <= 0 && u2 == 1
    y = u1;
else
    y = 0;
end
end

== matlab function VCU_CS75_12_16_Test/长安CS75底盘程序，20ms一次/APP/Controller/Longitudinal/MATLAB Function3 ==
  data: Ready input; RollingCounter output; LastCounter input
function RollingCounter   = fcn(Ready,LastCounter)
if LastCounter == 15
   RealCounter = 0;
else
   RealCounter = LastCounter; 
end

if Ready == 1
   RollingCounter = RealCounter + 1; 
else
   RollingCounter = RealCounter;
end
end

== matlab function VCU_CS75_12_16_Test/长安CS75底盘程序，20ms一次/APP/Controller/Longitudinal/MATLAB Function4 ==
  data: Ready input; RollingCounter output; LastCounter input
function RollingCounter   = fcn(Ready,LastCounter)
if LastCounter == 15
   RealCounter = 0;
else
   RealCounter = LastCounter; 
end

if Ready == 1
   RollingCounter = RealCounter + 1; 
else
   RollingCounter = RealCounter;
end
end

== matlab function VCU_CS75_12_16_Test/长安CS75底盘程序，20ms一次/APP/Controller/Longitudinal/MATLAB Function5 ==
  data: u1 input; y output; u2 input
function y = fcn(u1,u2)
if u2 >= 0 && u1 == 1
    y = u2;
else
    y = 0;
end
end

== matlab function VCU_CS75_12_16_Test/长安CS75底盘程序，20ms一次/APP/Controller/Longitudinal/MATLAB Function6 ==
  data: u input; y output
function y = fcn(u)
if u <= 0
    y = 0;
else
    y = 1;
end
end

== matlab function VCU_CS75_12_16_Test/长安CS75底盘程序，20ms一次/APP/Controller/Accesories/MATLAB Function ==
  data: u input; y1 output double; y2 output double
function [y1,y2] = fcn(u)
if u == 1
    y1 = 2;
    y2 = 2;
else
    y1 = 0;
    y2 = 0;
end
end

== matlab function VCU_CS75_12_16_Test/长安CS75底盘程序，20ms一次/APP/Controller/Accesories/MATLAB Function1 ==
  data: u1 input; y output; u2 input
function y = fcn(u1,u2)
if abs(u1-u2) == 1
    y = 1;  
else
    y = 0;
end
end

== matlab function VCU_CS75_12_16_Test/长安CS75底盘程序，20ms一次/Output/CAN0_Tx/to6004/MATLAB Function ==
  data: u input; y output
function y = fcn(u)
if u == 1
    y=0;
elseif u==2
    y=1;
elseif u==4;
    y=2;
else
    y=0;
end
end

== matlab function VCU_CS75_12_16_Test/长安CS75底盘程序，20ms一次/APP/Controller/Lateral/MATLAB Function1 ==
  data: L1 input; u1 input; y output; u2 input
function y = fcn(L1,u1,u2)
if (u1-u2)>L1
    y=u2+L1;
else
    if (u1-u2)<(-L1)
        y=u2-L1;
    else
        y=u1;
    end
end
end

== matlab function VCU_CS75_12_16_Test/长安CS75底盘程序，20ms一次/APP/Controller/Accesories/MATLAB Function2 ==
  data: u input; y output
function y = fcn(u)
if u == 1
    y = 1;
else
    y = 0;
end
end

== matlab function VCU_CS75_12_16_Test/长安CS75底盘程序，20ms一次/APP/Controller/Longitudinal/MATLAB Function7 ==
  data: u input; y output
function y = fcn(u)
if u == 1
    y = 1;
else
    y = 0;
end
end

== matlab function VCU_CS75_12_16_Test/长安CS75底盘程序，20ms一次/APP/Controller/Lateral/MATLAB Function7 ==
  data: u input; y output
function y = fcn(u)
if u == 1
    y = 1;
else
    y = 0;
end
end

== matlab function VCU_CS75_12_16_Test/长安CS75底盘程序，20ms一次/APP/Controller/Lateral/MATLAB Function ==
  data: LaterlAngleCommand input; SteeringTorqueOut output; Error output; SAS_SteeringAngle input; Ready input; ErrorSum output; P input; I input; D input; ErrorSumMax input; ErrorPre input; ErrorSumPre input
function [SteeringTorqueOut,Error,ErrorSum] = fcn(LaterlAngleCommand,SAS_SteeringAngle,Ready,P,I,D,ErrorSumMax,ErrorPre,ErrorSumPre)

Error = LaterlAngleCommand - SAS_SteeringAngle;%%%目标转角-当前转角，角度

if Ready == 1 
   ErrorSum = ErrorSumPre + Error;  %%累积误差 
else
   ErrorSum = 0;
end
%%%积分清零；

if ErrorSum > ErrorSumMax
    ErrorSum = ErrorSumMax;
elseif ErrorSum < -ErrorSumMax
    ErrorSum = -ErrorSumMax;
end
%%%积分限幅
    
PID_SteeringTorque = P*Error + I*ErrorSum + D*(Error - ErrorPre);
%%%位置式PID计算

if Ready == 1
    SteeringTorqueOut = PID_SteeringTorque; 
else
    SteeringTorqueOut = 0;
end
%%%实际的转矩输出

end

== matlab function VCU_CS75_12_16_Test/长安CS75底盘程序，20ms一次/Output/CAN0_Tx/to6001/MATLAB Function ==
  data: u1 input; y output; u2 input
function y = fcn(u1,u2)
if u2 == 0
    y = u1;
elseif u2 == 1
    y = -u1;
else
    y = 0;
end
end

== matlab function VCU_CS75_12_16_Test/长安CS75底盘程序，20ms一次/Output/CAN0_Tx/to6001/MATLAB Function1 ==
  data: u1 input; y output; u2 input
function y = fcn(u1,u2)
if u2 == 0
    y = u1;
elseif u2 == 1
    y = -u1;
else
    y = 0;
end
end

== matlab function VCU_CS75_12_16_Test/长安CS75底盘程序，20ms一次/Output/CAN0_Tx/to6001/MATLAB Function2 ==
  data: u1 input; y output; u2 input
function y = fcn(u1,u2)
if u2 == 0
    y = u1;
elseif u2 == 1
    y = -u1;
else
    y = 0;
end
end

== matlab function VCU_CS75_12_16_Test/长安CS75底盘程序，20ms一次/Output/CAN0_Tx/to6001/MATLAB Function3 ==
  data: u1 input; y output; u2 input
function y = fcn(u1,u2)
if u2 == 0
    y = u1;
elseif u2 == 1
    y = -u1;
else
    y = 0;
end
end

== matlab function VCU_CS75_12_16_Test/长安CS75底盘程序，20ms一次/Output/CAN0_Tx/to6002/MATLAB Function ==
  data: u input; y1 output; y2 output
function [y1,y2] = fcn(u)
if u <=0
    y1 = u;
    y2 = 0;
else
    y1 = 0;
    y2 = u;
end
end

== matlab function VCU_CS75_12_16_Test/长安CS75底盘程序，20ms一次/APP/Monitor/Vehicle_Status/MATLAB Function2 ==
  data: u1 input; y output; u2 input
function y = fcn(u1,u2)
if u1 == 1 || u2 ==1
    y = 1;
else
    y = 0;
end
end

== matlab function VCU_CS75_12_16_Test/长安CS75底盘程序，20ms一次/Input/CAN0_Rx/a1_211/ReceiveMessages/Subsystem/MATLAB Function1 ==
  data: u input; y output
function y = fcn(u)
y = u;
if u < 0
    y = u/20;
end
end

== matlab function VCU_CS75_12_16_Test/长安CS75底盘程序，20ms一次/APP/Controller/Lateral/MATLAB Function2 ==
  data: Ready input; RollingCounter output; LastCounter input
function RollingCounter   = fcn(Ready,LastCounter)
if LastCounter == 15
    RollingCounter = 0;
else
    if Ready == 1
        RollingCounter = LastCounter + 1;
    else
        RollingCounter = LastCounter; 
    end
end
end

== matlab function VCU_CS75_12_16_Test/长安CS75底盘程序，20ms一次/Input/ADC_Input/MATLAB Function ==
  data: u input; y output
function y = fcn(u)
if u == 1
    y = 0;
else
    y = 1;
end
end

== matlab function VCU_CS75_12_16_Test/长安CS75底盘程序，20ms一次/APP/Controller/Lateral/MATLAB Function4 ==
  data: T input; Tmax input; y output
function y = fcn(T,Tmax)
if T > Tmax
    y = Tmax;
elseif T < -Tmax
    y = -Tmax;
else
    y = T;
end
end
